simulink library "Flow_Mixer_basic"  (R2018b)
settings: Solver=ode45  StartTime=0.0  StopTime=10.0  RelTol=1e-3  EnableMultiTasking=on
undefined symbols (not defined in the file): DiameterLastPiece, DPConstant, DPLinear, DPQuadratic, FluidMix, FluidType, ID, MassFlow, Pressure, Temperature
libraries: carnot x1
settings Model: Creator=lena.frank  LastModifiedBy=P41573
settings DataIOCC: LimitDataPoints=on  SaveFormat=Array  SignalLoggingSaveFormat=ModelDataLogs
settings OptimizationCC: ExpressionDepthLimit=2147483647  LifeSpan=inf
settings DebuggingCC: UnderspecifiedInitializationDetection=Classic  MergeDetectMultiDrivingBlocksExec=none  SolverPrmCheckMsg=warning  FcnCallInpInsideContextMsg=warning  StateNameClashWarn=warning  SFUnexpectedBacktrackingDiag=warning  SFNoUnconditionalDefaultTransitionDiag=warning  SFExecutionAtInitializationDiag=none
settings HardwareCC: ProdBitPerPointer=32  ProdBitPerSizeT=32  ProdBitPerPtrDiffT=32  ProdLargestAtomicFloat=None  ProdIntDivRoundTo=Undefined  ProdEndianess=Unspecified  ProdWordSize=32  ProdHWDeviceType=32-bit Generic
settings ModelReferenceCC: PropagateSignalLabelsOutOfModel=off
settings SFSimCC: SimUseLocalCustomCode=off
settings RTWCC: RTWUseLocalCustomCode=off
settings CodeAppCC: StateflowObjectComments=on
settings GRTTargetCC: TargetLangStandard=C89/C90 (ANSI)  GeneratePreprocessorConditionals=Disable all  CombineOutputUpdateFcns=off  GRTInterface=on
settings ConfigComp: CovMetricSettings=dw  CovHtmlReporting=on  CovSaveCumulativeToWorkspaceVar=on  CovSaveSingleToWorkspaceVar=on  CovExternalEMLEnable=off

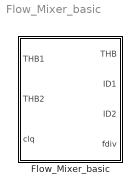
== system Flow_Mixer_basic ==
  Flow_Mixer_basic : Subsystem  mask(Flow Mixer Basic){}
      mask help:
      | The flow mixer calculated the temperature and massflow of 2 entering flows.
      | The temperature is calculated in the block Mix_T_Mdot.
      | The flow diversion fdiv (feed back to the flow diverter) takes care that the pressure drop in the 2 branches is the same. The resulting pressure drop coefficients are calulated in the s-function mix_flow (uses solve_quadratic_equation in Carlib).
      mask Help: web(fullfile(path_carnot('help'),'Flow_Mixer_basic.html'),'-helpbrowser')
      mask Display: disp('Flow\nMixer')

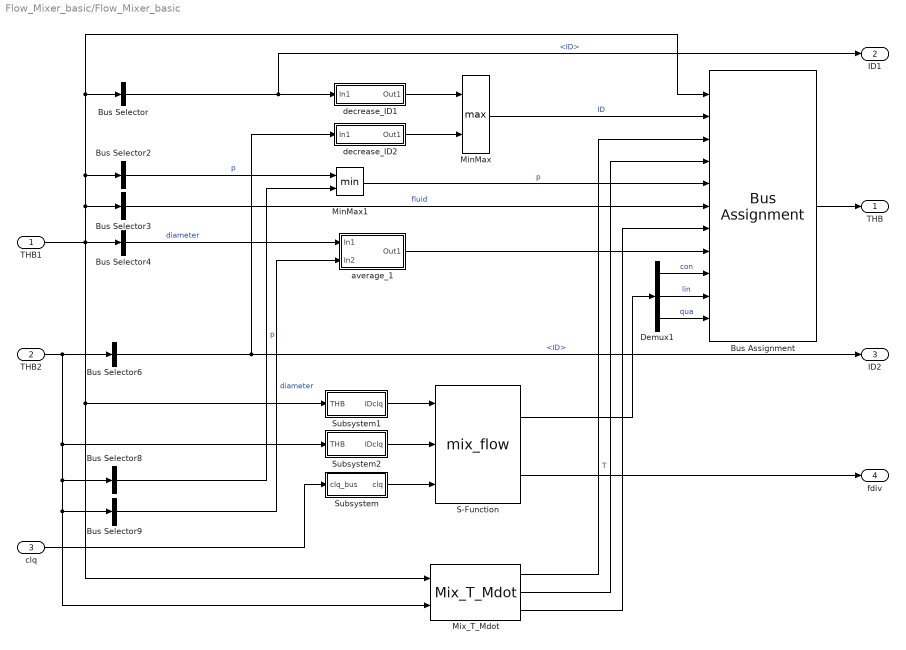
== system Flow_Mixer_basic/Flow_Mixer_basic ==
  THB1 : Inport
  THB2 : Inport  Port=2
  clq : Inport  Port=3
  Bus Assignment : BusAssignment  AssignedSignals=ID,Temperature,MassFlow,Pressure,FluidType,FluidMix,DiameterLastPiece,DPConstant,DPLinear,DPQuadratic
  Bus Selector : BusSelector  OutputSignals=ID
  Bus Selector2 : BusSelector  OutputSignals=Pressure  OutputAsBus=on
  Bus Selector3 : BusSelector  OutputSignals=FluidType  OutputAsBus=on
  Bus Selector4 : BusSelector  OutputSignals=DiameterLastPiece  OutputAsBus=on
  Bus Selector6 : BusSelector  OutputSignals=ID
  Bus Selector8 : BusSelector  OutputSignals=Pressure  OutputAsBus=on
  Bus Selector9 : BusSelector  OutputSignals=DiameterLastPiece  OutputAsBus=on
  Demux1 : Demux  Outputs=3
  MinMax : MinMax  Function=max  Inputs=2
  MinMax1 : MinMax  Inputs=2
  Mix_T_Mdot : carnot/Basic/Hydraulics/Mix_T_Mdot  mixcalc=Tmix = (mdot1*T1 + mdot2*T2)/(mdot1+mdot2)
      settings: SourceProductName=Carnot
  S-Function : S-Function  FunctionName=mix_flow  SFunctionDeploymentMode=off  EnableBusSupport=off
  Subsystem : Subsystem
  Subsystem1 : Subsystem
  Subsystem2 : Subsystem
  average_1 : Subsystem
  decrease_ID1 : Subsystem
  decrease_ID2 : Subsystem
  THB : Outport
  ID1 : Outport  Port=2
  ID2 : Outport  Port=3
  fdiv : Outport  Port=4
  wires:
  THB1/1 -> Bus Assignment/1, Bus Selector/1, Bus Selector2/1, Bus Selector3/1, Mix_T_Mdot/1, Subsystem1/1(THB), Bus Selector4/1
  Bus Selector/1 -> ID1/1, decrease_ID1/1(In1)  "<ID>"
  decrease_ID1/1(Out1) -> MinMax/1
  decrease_ID2/1(Out1) -> MinMax/2
  MinMax/1 -> Bus Assignment/2  "ID"
  Bus Selector3/1 -> Bus Assignment/6  "fluid"
  THB2/1 -> Mix_T_Mdot/2, Bus Selector9/1, Bus Selector8/1, Subsystem2/1(THB), Bus Selector6/1
  Bus Selector6/1 -> decrease_ID2/1(In1), ID2/1  "<ID>"
  Bus Selector8/1 -> MinMax1/2  "p"
  Bus Selector4/1 -> average_1/1(In1)  "diameter"
  Bus Selector9/1 -> average_1/2(In2)  "diameter"
  average_1/1(Out1) -> Bus Assignment/8
  MinMax1/1 -> Bus Assignment/5  "p"
  Demux1/1 -> Bus Assignment/9  "con"
  Demux1/2 -> Bus Assignment/10  "lin"
  Demux1/3 -> Bus Assignment/11  "qua"
  S-Function/1 -> Demux1/1
  Mix_T_Mdot/1 -> Bus Assignment/3  "T"
  Mix_T_Mdot/3 -> Bus Assignment/7
  Mix_T_Mdot/2 -> Bus Assignment/4
  Bus Selector2/1 -> MinMax1/1  "p"
  Subsystem2/1(IDclq) -> S-Function/2
  Bus Assignment/1 -> THB/1
  clq/1 -> Subsystem/1(clq_bus)
  S-Function/2 -> fdiv/1
  Subsystem/1(clq) -> S-Function/3
  Subsystem1/1(IDclq) -> S-Function/1

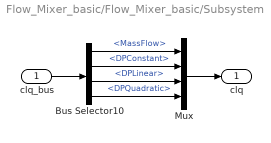
== system Flow_Mixer_basic/Flow_Mixer_basic/Subsystem ==
  clq_bus : Inport
  Bus Selector10 : BusSelector  OutputSignals=MassFlow,DPConstant,DPLinear,DPQuadratic
  Mux : Mux
  clq : Outport
  wires:
  Bus Selector10/1 -> Mux/1  "<MassFlow>"
  Bus Selector10/2 -> Mux/2  "<DPConstant>"
  Bus Selector10/3 -> Mux/3  "<DPLinear>"
  Bus Selector10/4 -> Mux/4  "<DPQuadratic>"
  clq_bus/1 -> Bus Selector10/1
  Mux/1 -> clq/1

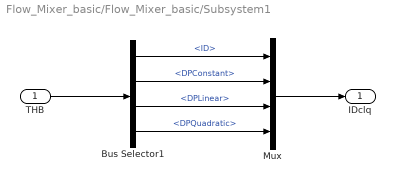
== system Flow_Mixer_basic/Flow_Mixer_basic/Subsystem1 ==
  THB : Inport
  Bus Selector1 : BusSelector  OutputSignals=ID,DPConstant,DPLinear,DPQuadratic
  Mux : Mux
  IDclq : Outport
  wires:
  THB/1 -> Bus Selector1/1
  Mux/1 -> IDclq/1
  Bus Selector1/1 -> Mux/1  "<ID>"
  Bus Selector1/2 -> Mux/2  "<DPConstant>"
  Bus Selector1/3 -> Mux/3  "<DPLinear>"
  Bus Selector1/4 -> Mux/4  "<DPQuadratic>"

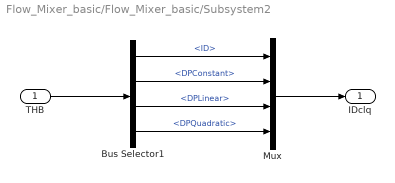
== system Flow_Mixer_basic/Flow_Mixer_basic/Subsystem2 ==
  THB : Inport
  Bus Selector1 : BusSelector  OutputSignals=ID,DPConstant,DPLinear,DPQuadratic
  Mux : Mux
  IDclq : Outport
  wires:
  Bus Selector1/4 -> Mux/4  "<DPQuadratic>"
  Bus Selector1/3 -> Mux/3  "<DPLinear>"
  Bus Selector1/2 -> Mux/2  "<DPConstant>"
  Bus Selector1/1 -> Mux/1  "<ID>"
  Mux/1 -> IDclq/1
  THB/1 -> Bus Selector1/1

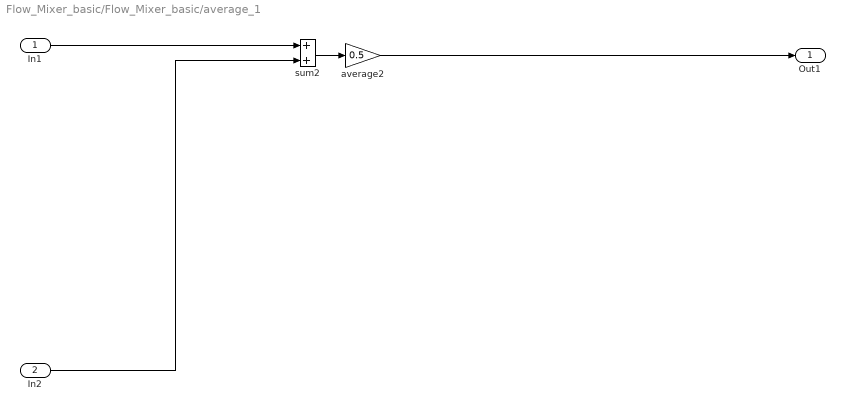
== system Flow_Mixer_basic/Flow_Mixer_basic/average_1 ==
  In1 : Inport
  In2 : Inport  Port=2
  average2 : Gain  Gain=0.5  SaturateOnIntegerOverflow=on  OutDataTypeStr=Inherit: Same as input  ParamDataTypeStr=Inherit: Same as input
  sum2 : Sum  SaturateOnIntegerOverflow=on  InputSameDT=on  OutDataTypeStr=Inherit: Same as first input
  Out1 : Outport
  wires:
  In2/1 -> sum2/2
  sum2/1 -> average2/1
  average2/1 -> Out1/1
  In1/1 -> sum2/1

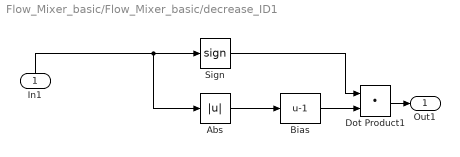
== system Flow_Mixer_basic/Flow_Mixer_basic/decrease_ID1 ==
  In1 : Inport
  Abs : Abs
  Bias : Bias  Bias=-1
  Dot Product1 : DotProduct  InputSameDT=on  OutDataTypeStr=Inherit: Inherit via internal rule
  Sign : Signum
  Out1 : Outport
  wires:
  In1/1 -> Abs/1, Sign/1
  Dot Product1/1 -> Out1/1
  Abs/1 -> Bias/1
  Sign/1 -> Dot Product1/1
  Bias/1 -> Dot Product1/2

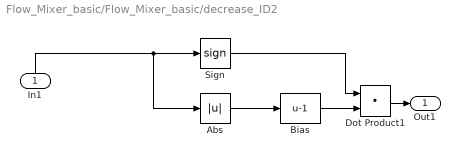
== system Flow_Mixer_basic/Flow_Mixer_basic/decrease_ID2 ==
  In1 : Inport
  Abs : Abs
  Bias : Bias  Bias=-1
  Dot Product1 : DotProduct  InputSameDT=on  OutDataTypeStr=Inherit: Inherit via internal rule
  Sign : Signum
  Out1 : Outport
  wires:
  Bias/1 -> Dot Product1/2
  Sign/1 -> Dot Product1/1
  Abs/1 -> Bias/1
  Dot Product1/1 -> Out1/1
  In1/1 -> Sign/1, Abs/1
